simulink model "buck"  (R2018a)
settings: Solver=VariableStepAuto  StartTime=0.0  StopTime=30e-3  MaxStep=1e-6  RelTol=1e-3  EnableMultiTasking=on
libraries: simulink x1
settings Model: Creator=Dilshan  LastModifiedBy=mahadi
settings DataIOCC: LimitDataPoints=on
settings OptimizationCC: LifeSpan=inf
settings DebuggingCC: AllowSymbolicDim=off  SFUnexpectedBacktrackingDiag=warning  SFNoUnconditionalDefaultTransitionDiag=warning  SFExecutionAtInitializationDiag=none
settings ModelReferenceCC: PropagateSignalLabelsOutOfModel=off
settings CodeAppCC: StateflowObjectComments=on
settings GRTTargetCC: TargetLangStandard=C89/C90 (ANSI)
settings ConfigComp: CovMetricSettings=dw  CovHtmlReporting=on  CovSaveCumulativeToWorkspaceVar=on  CovSaveSingleToWorkspaceVar=on  CovExternalEMLEnable=off
settings SimscapeCC: SimscapeNormalizeSystem=off
settings ConfigurationSet: Description=SimMechanics 2G

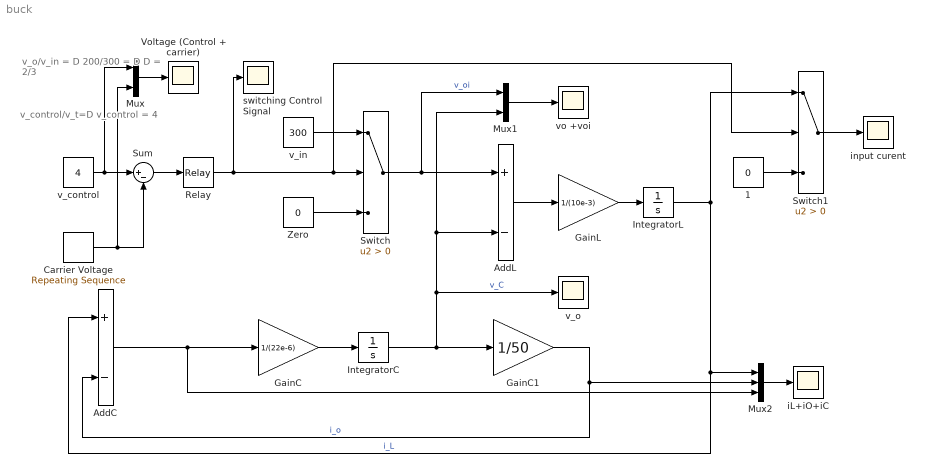
== system buck ==
  note: v_control/v_t=D
      | v_control = 4
  note: v_o/v_in = D
      | 200/300 = D
      | D = 2/3
  1 : Constant  Value=0
  AddC : Sum  Inputs=+-
  AddL : Sum  Inputs=+-
  Carrier Voltage : simulink/Sources/Repeating Sequence  rep_seq_t=[0 100e-6]  rep_seq_y=[0 6]
  GainC : Gain  Gain=1/(22e-6)
  GainC1 : Gain  Gain=1/50
  GainL : Gain  Gain=1/(10e-3)
  IntegratorC : Integrator
  IntegratorL : Integrator
  Mux : Mux  Inputs=2
  Mux1 : Mux  Inputs=2
  Mux2 : Mux  Inputs=3
  Relay : Relay
  Sum : Sum  Inputs=|+-
  Switch : Switch  Criteria=u2 > Threshold
  Switch1 : Switch  Criteria=u2 > Threshold
  Voltage (Control + carrier) : Scope
  Zero : Constant  Value=0
  iL+iO+iC : Scope
  input curent : Scope
  switching Control Signal : Scope
  v_control : Constant  Value=4
  v_in : Constant  Value=300
  v_o : Scope
  vo +voi : Scope
  wires:
  AddL/1 -> GainL/1
  GainL/1 -> IntegratorL/1
  IntegratorL/1 -> AddC/1, Mux2/1, Switch1/1  "i_L"
  Zero/1 -> Switch/3
  v_in/1 -> Switch/1
  Switch/1 -> Mux1/1, AddL/1  "v_oi"
  Relay/1 -> Switch1/2, Switch/2, switching Control Signal/1
  AddC/1 -> Mux2/3, GainC/1
  GainC/1 -> IntegratorC/1
  GainC1/1 -> Mux2/2, AddC/2  "i_o"
  IntegratorC/1 -> AddL/2, Mux1/2, v_o/1, GainC1/1  "v_C"
  v_control/1 -> Mux/1, Sum/1
  Carrier Voltage/1 -> Mux/2, Sum/2
  Sum/1 -> Relay/1
  Mux/1 -> Voltage (Control + carrier)/1
  Mux1/1 -> vo +voi/1
  Mux2/1 -> iL+iO+iC/1
  1/1 -> Switch1/3
  Switch1/1 -> input curent/1
